simulink model "send_cmd"  (R2021a)
settings: Solver=FixedStepAuto  StartTime=0.0  StopTime=inf  RelTol=1e-3
libraries: slrealtimesharedmemorylib x18, slrealtimeutilitieslib x3, slrealtimeiplib x1
settings Model: Creator=Ruixuan  LastModifiedBy=Ruixuan
settings SolverCC: ConcurrentTasks=on  PositivePriorityOrder=on  AutoInsertRateTranBlk=on  InsertRTBMode=Never (minimum delay)
settings OptimizationCC: BlockReduction=off  DefaultParameterBehavior=Inlined  OptimizeBlockIOStorage=off
settings DebuggingCC: TasksWithSamePriorityMsg=none
settings HardwareCC: ProdBitPerLong=64  ProdLongLongMode=on  ProdHWDeviceType=Intel->x86-64 (Linux 64)
settings ModelReferenceCC: ModelReferenceNumInstancesAllowed=Single
settings RTWCC: Description=Simulink Real-Time  SystemTargetFile=slrealtime.tlc  TemplateMakefile=slrealtime_default_tmf  Toolchain=Simulink Real-Time Toolchain  BuildConfiguration=Faster Runs  CodeExecutionProfiling=on  TargetLang=C++

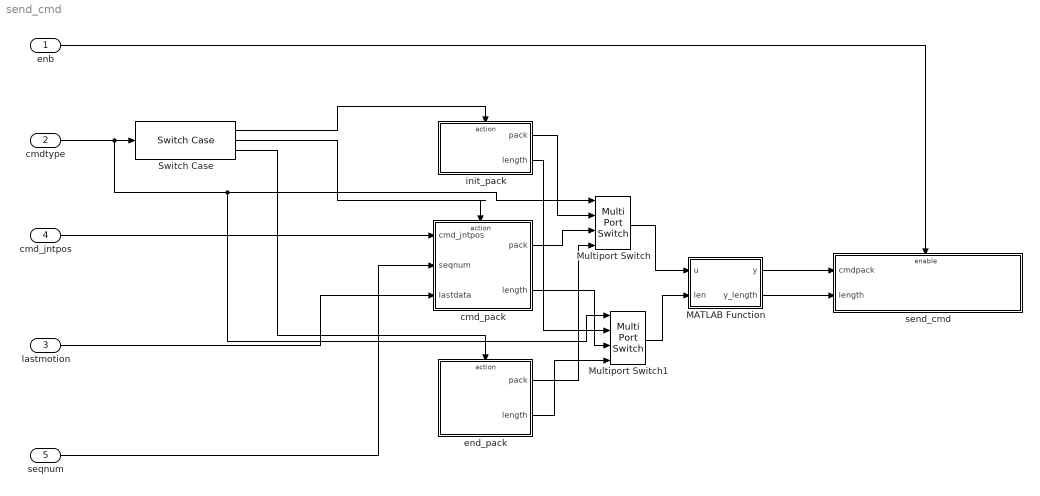
== system send_cmd ==
  enb : Inport
  cmdtype : Inport  Port=2
  lastmotion : Inport  Port=3
  cmd_jntpos : Inport  Port=4
  seqnum : Inport  Port=5
  MATLAB Function : MATLAB Function  TreatAsAtomicUnit=on
  Multiport Switch : MultiPortSwitch  DataPortOrder=Zero-based contiguous  zeroidx=on  AllowDiffInputSizes=on
  Multiport Switch1 : MultiPortSwitch  DataPortOrder=Zero-based contiguous  zeroidx=on
  Switch Case : SwitchCase  CaseConditions={0,1,2}  ShowDefaultCase=off
  cmd_pack : Subsystem
  end_pack : Subsystem
  init_pack : Subsystem  TreatAsAtomicUnit=on
  send_cmd : Subsystem
  wires:
  enb/1 -> send_cmd/Enable
  Switch Case/1 -> init_pack/Action
  Switch Case/2 -> cmd_pack/Action
  Multiport Switch/1 -> MATLAB Function/1(u)
  init_pack/1(pack) -> Multiport Switch/2
  cmd_pack/1(pack) -> Multiport Switch/3
  end_pack/1(pack) -> Multiport Switch/4
  Switch Case/3 -> end_pack/Action
  cmdtype/1 -> Multiport Switch/1, Multiport Switch1/1, Switch Case/1
  lastmotion/1 -> cmd_pack/3(lastdata)
  init_pack/2(length) -> Multiport Switch1/2
  cmd_jntpos/1 -> cmd_pack/1(cmd_jntpos)
  seqnum/1 -> cmd_pack/2(seqnum)
  cmd_pack/2(length) -> Multiport Switch1/3
  Multiport Switch1/1 -> MATLAB Function/2(len)
  end_pack/2(length) -> Multiport Switch1/4
  MATLAB Function/1(y) -> send_cmd/1(cmdpack)
  MATLAB Function/2(y_length) -> send_cmd/2(length)

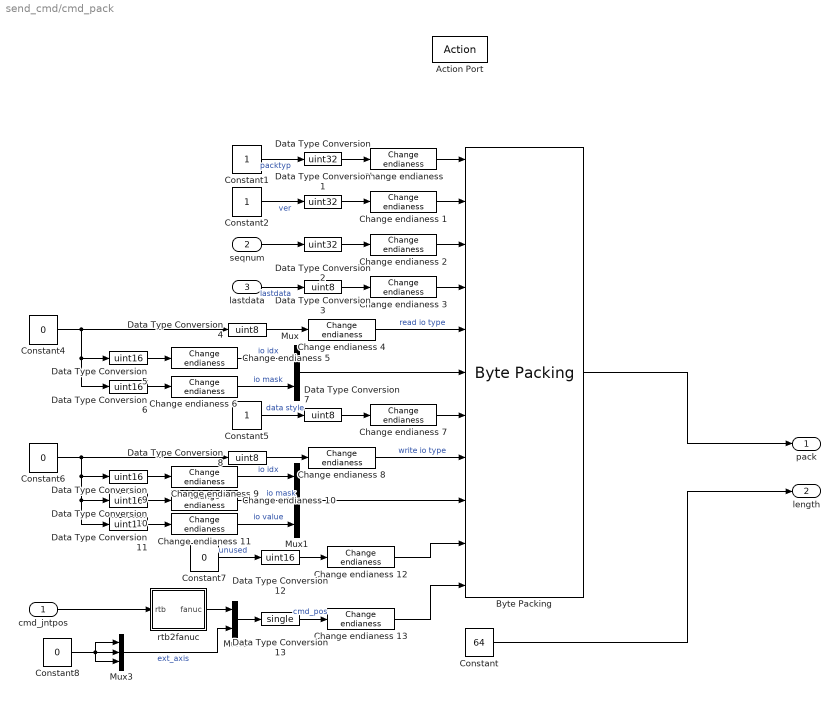
== system send_cmd/cmd_pack ==
  cmd_jntpos : Inport
  seqnum : Inport  Port=2
  lastdata : Inport  Port=3
  Action Port : ActionPort  ActionPortLabel=case [ 1 ]:
  "Byte Packing " : slrealtimeutilitieslib/Byte Packing  MaskPackedDataType=uint8  MaskUnpackedDataTypes={'uint32','uint32','uint32','uint8','uint8',['uint16'],'uint8','uint8',['uint16'],'uint16',['single']}  MaskAlignment=1
  Change endianess {,1..13} (14 alike) : slrealtimesharedmemorylib/Change endianess  numInp=1  lengthIn=Byte
      settings: SourceProductBaseCode=XP
  Constant : Constant  Value=64
  Constant1 : Constant
  Constant2 : Constant
  Constant{4,6..8} (4 alike) : Constant  Value=0
  Constant5 : Constant
  Data Type Conversion : DataTypeConversion  OutDataTypeStr=uint32
  Data Type Conversion1 : DataTypeConversion  OutDataTypeStr=uint32
  Data Type Conversion{5..6,9..12} (6 alike) : DataTypeConversion  OutDataTypeStr=uint16
  Data Type Conversion13 : DataTypeConversion  OutDataTypeStr=single
  Data Type Conversion2 : DataTypeConversion  OutDataTypeStr=uint32
  Data Type Conversion{3..4,7..8} (4 alike) : DataTypeConversion  OutDataTypeStr=uint8
  Mux : Mux  Inputs=2
  Mux1 : Mux  Inputs=3
  Mux2 : Mux  Inputs=[6,3]
  Mux3 : Mux  Inputs=3
  rtb2fanuc : Subsystem  mask(RTB2FANUC){}
      mask help: type convention from robotic toolbox style joint position to fanuc style joint position
  pack : Outport  VectorParamsAs1DForOutWhenUnconnected=off
  length : Outport  Port=2  VectorParamsAs1DForOutWhenUnconnected=off
  wires:
  Constant2/1 -> Data Type Conversion1/1  "ver"
  Change endianess 1/1 -> "Byte Packing "/2
  Data Type Conversion/1 -> "Change endianess "/1
  Constant1/1 -> Data Type Conversion/1  "packtyp"
  "Change endianess "/1 -> "Byte Packing "/1
  Data Type Conversion1/1 -> Change endianess 1/1
  seqnum/1 -> Data Type Conversion2/1
  Change endianess 2/1 -> "Byte Packing "/3
  Data Type Conversion2/1 -> Change endianess 2/1
  lastdata/1 -> Data Type Conversion3/1  "lastdata"
  Change endianess 3/1 -> "Byte Packing "/4
  Data Type Conversion3/1 -> Change endianess 3/1
  Data Type Conversion4/1 -> Change endianess 4/1
  Change endianess 4/1 -> "Byte Packing "/5  "read io type"
  Data Type Conversion5/1 -> Change endianess 5/1
  Data Type Conversion6/1 -> Change endianess 6/1
  Change endianess 5/1 -> Mux/1  "io idx"
  Change endianess 6/1 -> Mux/2  "io mask"
  Constant4/1 -> Data Type Conversion4/1, Data Type Conversion5/1, Data Type Conversion6/1
  Mux/1 -> "Byte Packing "/6
  Data Type Conversion7/1 -> Change endianess 7/1
  Constant5/1 -> Data Type Conversion7/1  "data style"
  Change endianess 7/1 -> "Byte Packing "/7
  Mux1/1 -> "Byte Packing "/9
  Data Type Conversion10/1 -> Change endianess 10/1
  Change endianess 10/1 -> Mux1/2  "io mask"
  Data Type Conversion9/1 -> Change endianess 9/1
  Constant6/1 -> Data Type Conversion8/1, Data Type Conversion9/1, Data Type Conversion11/1, Data Type Conversion10/1
  Change endianess 9/1 -> Mux1/1  "io idx"
  Data Type Conversion8/1 -> Change endianess 8/1
  Change endianess 8/1 -> "Byte Packing "/8  "write io type"
  Data Type Conversion11/1 -> Change endianess 11/1
  Change endianess 11/1 -> Mux1/3  "io value"
  Data Type Conversion12/1 -> Change endianess 12/1
  Constant7/1 -> Data Type Conversion12/1  "unused"
  Change endianess 12/1 -> "Byte Packing "/10
  cmd_jntpos/1 -> rtb2fanuc/1(rtb)
  rtb2fanuc/1(fanuc) -> Mux2/1
  Mux3/1 -> Mux2/2  "ext_axis"
  Constant8/1 -> Mux3/3, Mux3/2, Mux3/1
  Mux2/1 -> Data Type Conversion13/1
  Change endianess 13/1 -> "Byte Packing "/11
  "Byte Packing "/1 -> pack/1
  Constant/1 -> length/1
  Data Type Conversion13/1 -> Change endianess 13/1  "cmd_pos"

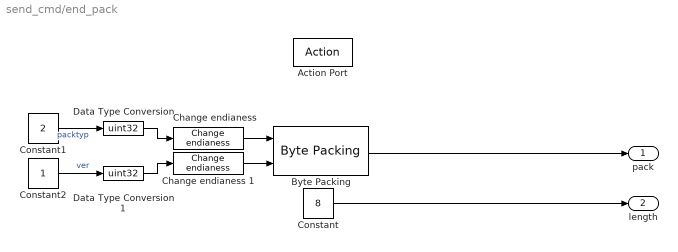
== system send_cmd/end_pack ==
  Action Port : ActionPort  ActionPortLabel=case [ 2 ]:
  "Byte Packing " : slrealtimeutilitieslib/Byte Packing  MaskPackedDataType=uint8  MaskUnpackedDataTypes={'uint32','uint32'}  MaskAlignment=1
  "Change endianess " : slrealtimesharedmemorylib/Change endianess  numInp=1  lengthIn=Byte
      settings: SourceProductBaseCode=XP
  Change endianess 1 : slrealtimesharedmemorylib/Change endianess  numInp=1  lengthIn=Byte
      settings: SourceProductBaseCode=XP
  Constant : Constant  Value=8
  Constant1 : Constant  Value=2
  Constant2 : Constant
  Data Type Conversion : DataTypeConversion  OutDataTypeStr=uint32
  Data Type Conversion1 : DataTypeConversion  OutDataTypeStr=uint32
  pack : Outport  VectorParamsAs1DForOutWhenUnconnected=off
  length : Outport  Port=2  VectorParamsAs1DForOutWhenUnconnected=off
  wires:
  Constant2/1 -> Data Type Conversion1/1  "ver"
  Change endianess 1/1 -> "Byte Packing "/2
  Data Type Conversion/1 -> "Change endianess "/1
  Constant1/1 -> Data Type Conversion/1  "packtyp"
  "Change endianess "/1 -> "Byte Packing "/1
  Data Type Conversion1/1 -> Change endianess 1/1
  "Byte Packing "/1 -> pack/1
  Constant/1 -> length/1

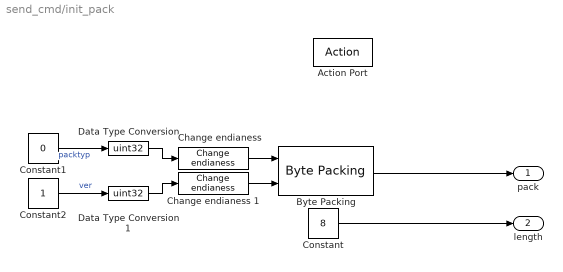
== system send_cmd/init_pack ==
  Action Port : ActionPort  ActionPortLabel=case [ 0 ]:
  "Byte Packing " : slrealtimeutilitieslib/Byte Packing  MaskPackedDataType=uint8  MaskUnpackedDataTypes={'uint32','uint32'}  MaskAlignment=1
  "Change endianess " : slrealtimesharedmemorylib/Change endianess  numInp=1  lengthIn=Byte
      settings: SourceProductBaseCode=XP
  Change endianess 1 : slrealtimesharedmemorylib/Change endianess  numInp=1  lengthIn=Byte
      settings: SourceProductBaseCode=XP
  Constant : Constant  Value=8
  Constant1 : Constant  Value=0
  Constant2 : Constant
  Data Type Conversion : DataTypeConversion  OutDataTypeStr=uint32
  Data Type Conversion1 : DataTypeConversion  OutDataTypeStr=uint32
  pack : Outport  VectorParamsAs1DForOutWhenUnconnected=off
  length : Outport  Port=2  VectorParamsAs1DForOutWhenUnconnected=off
  wires:
  Data Type Conversion/1 -> "Change endianess "/1
  "Change endianess "/1 -> "Byte Packing "/1
  Data Type Conversion1/1 -> Change endianess 1/1
  Constant1/1 -> Data Type Conversion/1  "packtyp"
  Change endianess 1/1 -> "Byte Packing "/2
  Constant2/1 -> Data Type Conversion1/1  "ver"
  "Byte Packing "/1 -> pack/1
  Constant/1 -> length/1

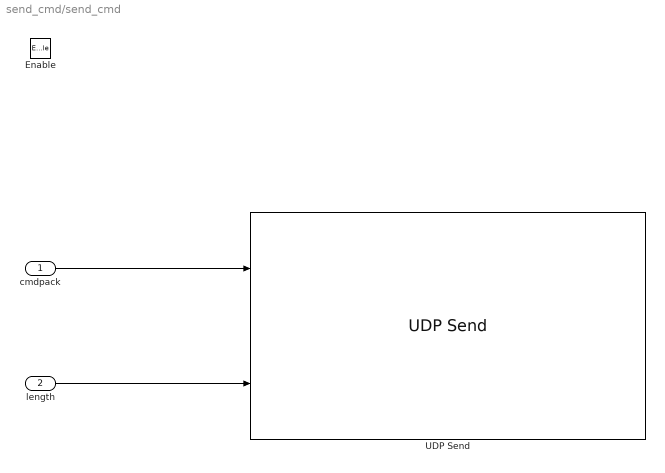
== system send_cmd/send_cmd ==
  cmdpack : Inport
  length : Inport  Port=2
  Enable : EnablePort
  UDP Send : slrealtimeiplib/UDP Send  useHostTargetConn=off  ipAddress=192.168.1.101  localPort=60015  toAddress=192.168.1.100  toPort=60015  sampleTime=Ts
      settings: SourceProductBaseCode=XP
  wires:
  length/1 -> UDP Send/2
  cmdpack/1 -> UDP Send/1

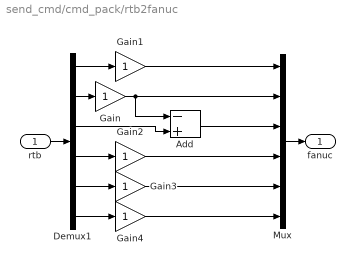
== system send_cmd/cmd_pack/rtb2fanuc ==
  rtb : Inport
  Add : Sum  Inputs=-+
  Demux1 : Demux  Outputs=6
  Gain{,1..4} (5 alike) : Gain
  Mux : Mux  Inputs=6
  fanuc : Outport  VectorParamsAs1DForOutWhenUnconnected=off
  wires:
  Demux1/3 -> Add/2
  Demux1/2 -> Gain/1
  Gain/1 -> Mux/2, Add/1
  Add/1 -> Mux/3
  Demux1/6 -> Gain4/1
  Demux1/1 -> Gain1/1
  Demux1/5 -> Gain3/1
  Demux1/4 -> Gain2/1
  Mux/1 -> fanuc/1
  rtb/1 -> Demux1/1
  Gain1/1 -> Mux/1
  Gain2/1 -> Mux/4
  Gain3/1 -> Mux/5
  Gain4/1 -> Mux/6

== matlab function send_cmd/MATLAB Function ==
  data: u input; y output; y_length output; len input
function [y,y_length] = fcn(u,len)
y = uint8(zeros(132,1));
y_length = len;
for a = 1:y_length
    y(a) = u(a);
end
